simulink model "model1"  (R2021b)
settings: Solver=VariableStepAuto  StartTime=0.0  StopTime=10.0  RelTol=1e-3
libraries: simulink x8
settings Model: SimulationMode=accelerator  Creator=O  LastModifiedBy=user2

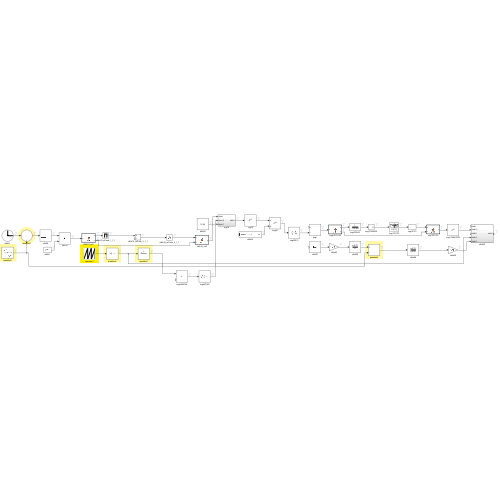
[thumbnail: Simulink's stored preview of the top-level diagram]
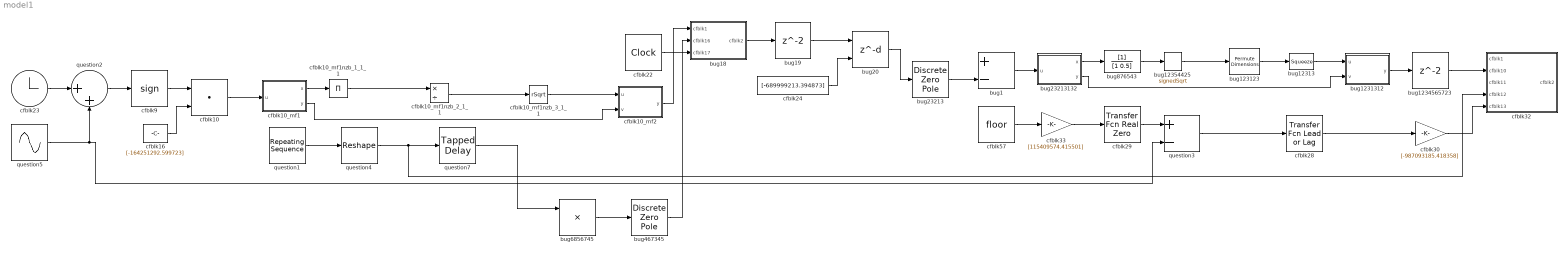
== system model1 ==
  bug1 : Sum  Inputs=+-  OutDataTypeStr=double
  bug123123 : PermuteDimensions
  bug12313 : Squeeze
  bug1231312 : MATLAB Function  TreatAsAtomicUnit=on
  bug1234565723 : Delay  SampleTime=1
  bug12354425 : Sqrt  Operator=signedSqrt  SaturateOnIntegerOverflow=on
  bug18 : Subsystem
  bug19 : Delay  SampleTime=1
  bug20 : Delay  DelayLengthSource=Input port  SampleTime=1
      settings: InputPortMap=u0,p1
  bug23213 : DiscreteZeroPole  Poles=[0 0.5]  Gain=1
  bug23213132 : MATLAB Function  TreatAsAtomicUnit=on
  bug467345 : DiscreteZeroPole  Poles=[0 0.5]  Gain=1
  bug6856745 : Product  Inputs=**  OutDataTypeStr=double
  bug876543 : DiscreteFilter
  cfblk10 : DotProduct  OutDataTypeStr=double  InputSameDT=on
  cfblk10_mf1 : MATLAB Function  TreatAsAtomicUnit=on
  cfblk10_mf1nzb_1_1_1 : Product  Inputs=*
  cfblk10_mf1nzb_2_1_1 : Product  Inputs=*/
  cfblk10_mf1nzb_3_1_1 : Sqrt  Operator=rSqrt  SaturateOnIntegerOverflow=on
  cfblk10_mf2 : MATLAB Function  TreatAsAtomicUnit=on
  cfblk16 : Constant  Value=[-164251292.599723]  OutDataTypeStr=double  SampleTime=1
  cfblk22 : DigitalClock
  cfblk23 : Clock
  cfblk24 : Constant  Value=[-689999213.394873]  OutDataTypeStr=double  SampleTime=1
  cfblk28 : simulink/Discrete/Transfer Fcn Lead or Lag  PoleZ=0.95  ZeroZ=0.75  ICPrevOutput=0.0  ICPrevInput=0.0  DoSatur=off
      settings: SourceProductBaseCode=SL
  cfblk29 : simulink/Discrete/Transfer Fcn Real Zero  ZeroZ=0.75  ICPrevInput=0.0  DoSatur=off
      settings: SourceProductBaseCode=SL
  cfblk30 : Gain  Gain=[-987093185.418358]  OutDataTypeStr=double
  cfblk32 : Subsystem
  cfblk33 : Gain  Gain=[115409574.415501]  OutDataTypeStr=double
  cfblk57 : Rounding
  cfblk9 : Signum
  question1 : simulink/Sources/Repeating Sequence  rep_seq_t=[0 2]  rep_seq_y=[-336118232.963542, 705195365.662670]
  question2 : Sum  Inputs=|++  OutDataTypeStr=double
  question3 : Sum  Inputs=+-  OutDataTypeStr=double
  question4 : Reshape
  question5 : Sin  Amplitude=[135374790.730569]  Bias=[-517354260.574814]  SampleTime=0
  question7 : simulink/Discrete/Tapped Delay  vinit=0.0  samptime=-1  NumDelays=1  DelayOrder=Oldest  includeCurrent=off
  wires:
  cfblk29/1 -> question3/1
  question3/1 -> cfblk28/1
  cfblk28/1 -> cfblk30/1
  cfblk33/1 -> cfblk29/1
  cfblk10_mf1/1(x) -> cfblk10_mf1nzb_1_1_1/1
  cfblk57/1 -> cfblk33/1
  question4/1 -> question7/1, cfblk32/4(cfblk12)
  question1/1 -> question4/1
  cfblk22/1 -> bug18/3(cfblk17)
  cfblk9/1 -> cfblk10/1
  bug1/1 -> bug23213132/1(u)
  question2/1 -> cfblk9/1
  bug23213132/1(x) -> bug876543/1
  cfblk10_mf1nzb_2_1_1/1 -> cfblk10_mf1nzb_3_1_1/1
  cfblk10_mf1nzb_3_1_1/1 -> cfblk10_mf2/1(u)
  cfblk10_mf1nzb_1_1_1/1 -> cfblk10_mf1nzb_2_1_1/1
  cfblk10_mf1/2(y) -> cfblk10_mf2/2(v)
  cfblk10/1 -> cfblk10_mf1/1(u)
  bug123123/1 -> bug12313/1
  bug23213/1 -> bug1/2
  bug1231312/1(y) -> bug1234565723/1
  bug19/1 -> bug20/1
  cfblk30/1 -> cfblk32/5(cfblk13)
  bug23213132/2(y) -> bug1231312/2(v)
  bug876543/1 -> bug12354425/1
  cfblk10_mf2/1(y) -> bug18/1(cfblk1)
  bug1234565723/1 -> cfblk32/2(cfblk10)
  bug18/1(cfblk2) -> bug19/1
  question7/1 -> bug6856745/1
  question5/1 -> question2/2, question3/2
  bug6856745/1 -> bug467345/1
  cfblk24/1 -> bug20/2
  bug467345/1 -> bug18/2(cfblk16)
  bug20/1 -> bug23213/1
  bug12313/1 -> bug1231312/1(u)
  bug12354425/1 -> bug123123/1
  cfblk23/1 -> question2/1
  cfblk16/1 -> cfblk10/2

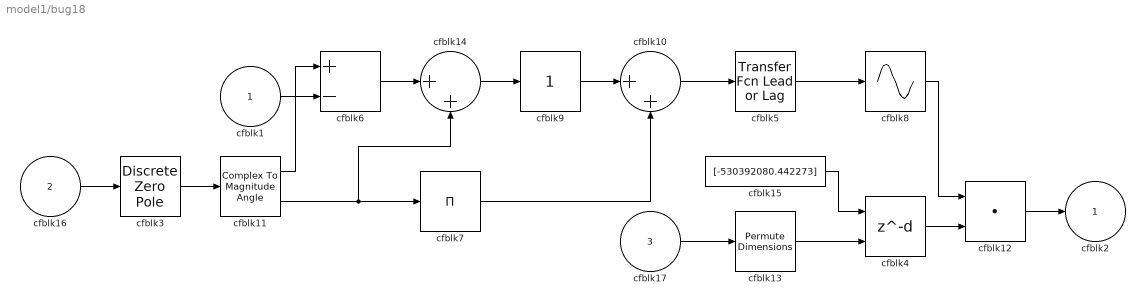
== system model1/bug18 ==
  cfblk1 : Inport
  cfblk16 : Inport  Port=2
  cfblk17 : Inport  Port=3
  cfblk10 : Sum  Inputs=|++  OutDataTypeStr=double
  cfblk11 : ComplexToMagnitudeAngle
  cfblk12 : DotProduct  OutDataTypeStr=double  InputSameDT=on
  cfblk13 : PermuteDimensions
  cfblk14 : Sum  Inputs=|++  OutDataTypeStr=double
  cfblk15 : Constant  Value=[-530392080.442273]  OutDataTypeStr=double  SampleTime=1
  cfblk3 : DiscreteZeroPole  Poles=[0 0.5]  Gain=1
  cfblk4 : Delay  DelayLengthSource=Input port  SampleTime=1
      settings: InputPortMap=u0,p1
  cfblk5 : simulink/Discrete/Transfer Fcn Lead or Lag  PoleZ=0.95  ZeroZ=0.75  ICPrevOutput=0.0  ICPrevInput=0.0  DoSatur=off
      settings: SourceProductBaseCode=SL
  cfblk6 : Sum  Inputs=+-  OutDataTypeStr=double
  cfblk7 : Product  Inputs=*  OutDataTypeStr=double
  cfblk8 : Sin  TimeSource=Use external signal  SampleTime=0
  cfblk9 : simulink/Math Operations/Slider Gain  gain=1  low=0  high=2
  cfblk2 : Outport
  wires:
  cfblk7/1 -> cfblk10/2
  cfblk15/1 -> cfblk4/1
  cfblk8/1 -> cfblk12/1
  cfblk14/1 -> cfblk9/1
  cfblk4/1 -> cfblk12/2
  cfblk5/1 -> cfblk8/1
  cfblk12/1 -> cfblk2/1
  cfblk11/1 -> cfblk6/1
  cfblk10/1 -> cfblk5/1
  cfblk16/1 -> cfblk3/1
  cfblk13/1 -> cfblk4/2
  cfblk1/1 -> cfblk6/2
  cfblk3/1 -> cfblk11/1
  cfblk17/1 -> cfblk13/1
  cfblk6/1 -> cfblk14/1
  cfblk9/1 -> cfblk10/1
  cfblk11/2 -> cfblk7/1, cfblk14/2

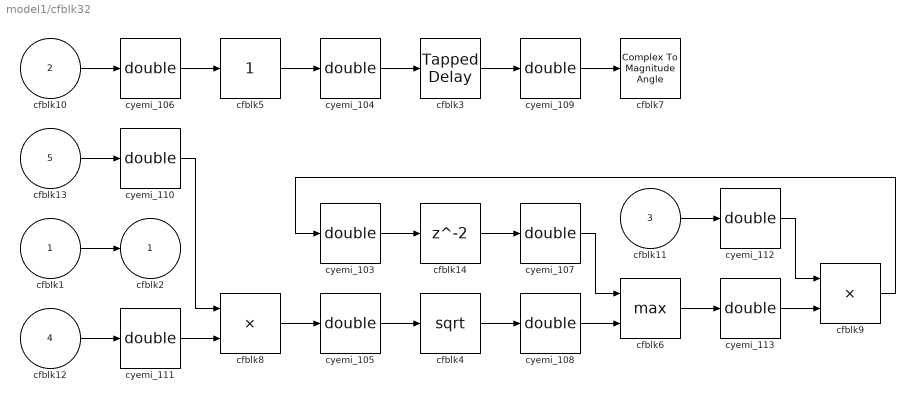
== system model1/cfblk32 ==
  cfblk1 : Inport
  cfblk10 : Inport  Port=2
  cfblk11 : Inport  Port=3
  cfblk12 : Inport  Port=4
  cfblk13 : Inport  Port=5
  cfblk14 : Delay  SampleTime=1
  cfblk3 : simulink/Discrete/Tapped Delay  vinit=0.0  samptime=-1  NumDelays=1  DelayOrder=Oldest  includeCurrent=off
  cfblk4 : Sqrt  OutDataTypeStr=double  SaturateOnIntegerOverflow=on
  cfblk5 : simulink/Math Operations/Slider Gain  gain=1  low=0  high=2
  cfblk6 : MinMax  Function=max  Inputs=2  OutDataTypeStr=double
  cfblk7 : ComplexToMagnitudeAngle
  cfblk8 : Product  OutDataTypeStr=double
  cfblk9 : Product  OutDataTypeStr=double
  cyemi_{103..113} (11 alike) : DataTypeConversion  OutDataTypeStr=double
  cfblk2 : Outport
  wires:
  cyemi_106/1 -> cfblk5/1
  cyemi_110/1 -> cfblk8/1
  cfblk9/1 -> cyemi_103/1
  cfblk4/1 -> cyemi_108/1
  cfblk13/1 -> cyemi_110/1
  cyemi_108/1 -> cfblk6/2
  cfblk11/1 -> cyemi_112/1
  cyemi_111/1 -> cfblk8/2
  cyemi_104/1 -> cfblk3/1
  cyemi_113/1 -> cfblk9/2
  cfblk12/1 -> cyemi_111/1
  cyemi_105/1 -> cfblk4/1
  cyemi_107/1 -> cfblk6/1
  cyemi_112/1 -> cfblk9/1
  cfblk8/1 -> cyemi_105/1
  cfblk3/1 -> cyemi_109/1
  cfblk6/1 -> cyemi_113/1
  cfblk10/1 -> cyemi_106/1
  cfblk14/1 -> cyemi_107/1
  cyemi_109/1 -> cfblk7/1
  cfblk1/1 -> cfblk2/1
  cyemi_103/1 -> cfblk14/1
  cfblk5/1 -> cyemi_104/1

== matlab function model1/cfblk10_mf2 ==
  data: u input; y output; v input
function y = mf2(u,v)
u = v;
y = u;
end

== matlab function model1/bug23213132 ==
  data: x output; u input; y output
function [x,y]= mf1(u)
x = u;
y = u;
end

== matlab function model1/bug1231312 ==
  data: u input; y output; v input
function y = mf2(u,v)
u = v;
y = u;
end

== matlab function model1/cfblk10_mf1 ==
  data: x output; u input; y output
function [x,y]= mf1(u)
x = u;
y = u;
end
